simulink model "graphmake"  (R2020a)
settings: Solver=VariableStepAuto  StartTime=0.0  StopTime=10.0  RelTol=1e-3
settings Model: Creator=Jason  LastModifiedBy=Jason

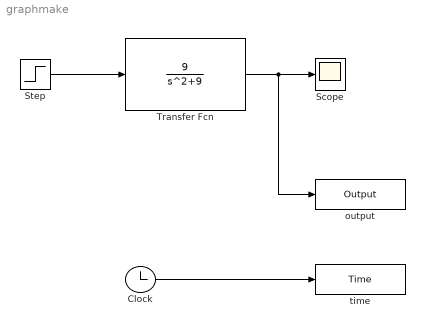
== system graphmake ==
  Clock : Clock
  Scope : Scope
  Step : Step  SampleTime=0
  Transfer Fcn : TransferFcn  Numerator=[9]  Denominator=[1 0 9]
  output : ToWorkspace  VariableName=Output  SampleTime=-1
  time : ToWorkspace  VariableName=Time  SampleTime=-1
  wires:
  Step/1 -> Transfer Fcn/1
  Transfer Fcn/1 -> output/1, Scope/1
  Clock/1 -> time/1
